simulink model "kalman_scattering_based_fv"  (R2020b)
settings: Solver=ode45  StartTime=0.0  StopTime=30  RelTol=1e-3
values from neighbouring files (symbols this model uses):
  A = [1 Ts ... (first row only)    [kalman_hw6_main_fv.m]
  Amp = 0.3    [kalman_hw6_main_fv.m]
  b = 1    [kalman_hw6_main_fv.m]
  Be = 20    [kalman_hw6_main_fv.m]
  Bh = 1.5    [kalman_hw6_main_fv.m]
  Bs = 50    [kalman_hw6_main_fv.m]
  C = [1 0]    [kalman_hw6_main_fv.m]
  delay = 10    [kalman_hw6_main_fv.m]
  Dh = 8    [kalman_hw6_main_fv.m]
  Dm = 0    [kalman_hw6_main_fv.m]
  Ds = 0    [kalman_hw6_main_fv.m]
  Fc_lp = 5    [kalman_hw6_main_fv.m]
  Fc_sin = 0.1    [kalman_hw6_main_fv.m]
  Fc_wave = 8    [kalman_hw6_main_fv.m]
  Je = 0    [kalman_hw6_main_fv.m]
  Jh = 0    [kalman_hw6_main_fv.m]
  Ke = 210    [kalman_hw6_main_fv.m]
  Kh = 0.1    [kalman_hw6_main_fv.m]
  Ks = 60    [kalman_hw6_main_fv.m]
  Mm = 0.5    [kalman_hw6_main_fv.m]
  Ms = 2    [kalman_hw6_main_fv.m]
  Ph = 1    [kalman_hw6_main_fv.m]
  posNoiseVar = 0.0001    [kalman_hw6_main_fv.m]
  R_m = 1    [kalman_hw6_main_fv.m]
  R_s = 1    [kalman_hw6_main_fv.m]
  torqueNoiseVar = 0.01    [kalman_hw6_main_fv.m]
  Ts = 0.001    [kalman_hw6_main_fv.m]
  xe = 0.5    [kalman_hw6_main_fv.m]
undefined symbols (not defined in the file or in its folder): DiscIntNeverNeededParam, Discrete, Time
libraries: simulink x4, ctrlSharedLib x2
settings Model: Creator=nicol  LastModifiedBy=nicol

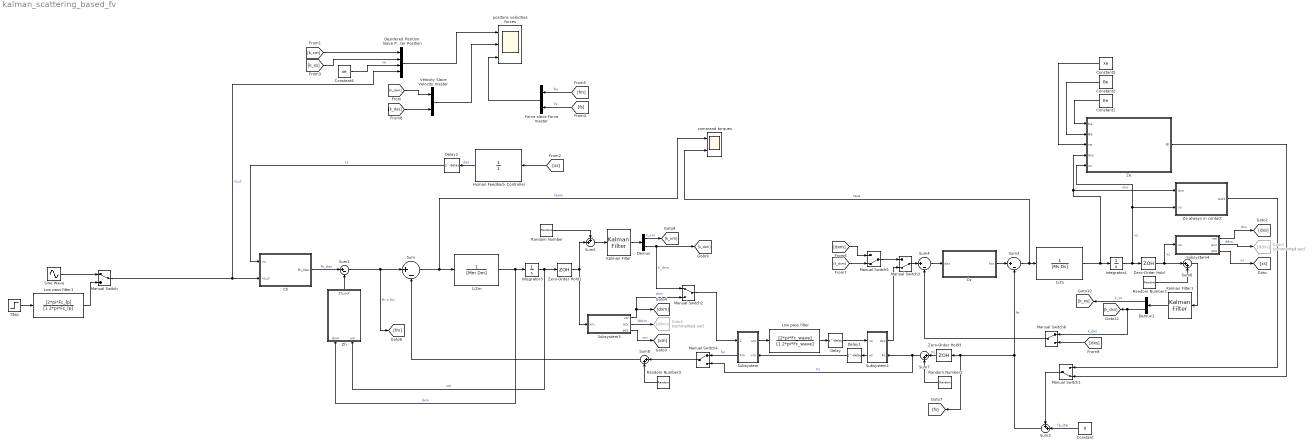
== system kalman_scattering_based_fv ==
  1/Zm : TransferFcn  Denominator=[Mm Dm]
  1/Zs : TransferFcn  Denominator=[Ms Ds]
  Ch : Subsystem
  Constant : Constant  Value=0
  Constant1 : Constant  Value=Ke
  Constant2 : Constant  Value=Be
  Constant3 : Constant  Value=xe
  Constant4 : Constant  Value=xe
  Cs : Subsystem
  Delay : Delay  DelayLength=delay  SampleTime=Ts
  Delay1 : Delay  DelayLength=delay  SampleTime=Ts
  Delay2 : Delay  DelayLength=delay  SampleTime=Ts
  Demux : Demux  Outputs=2
  Demux1 : Demux  Outputs=2
  Desidered Position Slave Position Master Position : Mux
  Force slave Force master : Mux  Inputs=2
  Goto2 : Goto  Commented=on  GotoTag=ddxs
  Goto5 : Goto  Commented=on  GotoTag=ddxm
  Human Feedback Controller : TransferFcn  Denominator=[1]
  Integrator3 : Integrator
  Integrator4 : Integrator
  Kalman Filter : ctrlSharedLib/Kalman Filter  TimeDomain=Discrete-Time  UseCurrentEstimator=on  ModelSource=Individual A, B, C, D matrices  ModelSourceVariable=ss(0.95,1,0,0,Ts)  A=A  B=1  C=C  D=0  NumberOfStates=1  NumberOfInputs=1  NumberOfOutputs=1  InitialEstimateSource=Dialog  X0=0  P0=10  UseK=off  UseGH=off  NumberOfProcessNoiseInputs=1  G=1  TimeInvariantG=on  H=0  TimeInvariantH=on  Q=Q_m  TimeInvariantQ=on  R=R_m  TimeInvariantR=on  N=0  TimeInvariantN=on  AddInputPort=off  AddEnablePort=off  OutputEstimatedY=off  OutputP=off  Ts=Ts
  Kalman Filter1 : ctrlSharedLib/Kalman Filter  TimeDomain=Discrete-Time  UseCurrentEstimator=on  ModelSource=Individual A, B, C, D matrices  ModelSourceVariable=ss(0.95,1,0,0,Ts)  A=A  B=1  C=C  D=0  NumberOfStates=1  NumberOfInputs=1  NumberOfOutputs=1  InitialEstimateSource=Dialog  X0=0  P0=10  UseK=off  UseGH=off  NumberOfProcessNoiseInputs=1  G=1  TimeInvariantG=on  H=0  TimeInvariantH=on  Q=Q_s  TimeInvariantQ=on  R=R_s  TimeInvariantR=on  N=0  TimeInvariantN=on  AddInputPort=off  AddEnablePort=off  OutputEstimatedY=off  OutputP=off  Ts=Ts
  Low pass filter : TransferFcn  Numerator=[2*pi*Fc_wave]  Denominator=[1 2*pi*Fc_wave]
  Low pass filter1 : TransferFcn  Numerator=[2*pi*Fc_lp]  Denominator=[1 2*pi*Fc_lp]
  Manual Switch{,2,4,6} (4 alike) : ManualSwitch
  Manual Switch1 : ManualSwitch  CurrentSetting=0
  Manual Switch3 : ManualSwitch  CurrentSetting=0
  Manual Switch5 : ManualSwitch  CurrentSetting=0
  Random Number : RandomNumber  Variance=posNoiseVar  SampleTime=Ts
  Random Number1 : RandomNumber  Variance=posNoiseVar  SampleTime=Ts
  Random Number2 : RandomNumber  Variance=torqueNoiseVar  SampleTime=Ts
  Random Number3 : RandomNumber  Variance=torqueNoiseVar  SampleTime=Ts
  Sine Wave : Sin  Amplitude=Amp  Frequency=2*pi*Fc_sin  SampleTime=0
  Step : Step  Time=Amp  After=Amp  SampleTime=0
  Subsystem : Subsystem
      settings: PortSchema="{\"entries\":[{\"content\":{\"sides\":[{\"content\":{\"connectorIds\":[\"In1\",\"Out2\"]},\"type\":\"ConnectorPlacement.EquallySpacedRectSide\",\"uuid\":\"82be490b-f4e1-4469-8bd6-488a0e070f91\"},{\"content\":{\"connectorIds\":[\"Out1\",\"In2\"],\"side\":\"RIGHT\"},\"type\":\"ConnectorPlacement.EquallySpacedRectSide\",\"uuid\":\"c4a13bf6-21c5-475e-be70-cb3636e820b8\"},{\"content\":{\"connectorIds\":[],\"side\":\"TOP\"},\"type\":\"ConnectorPlacement.EquallySpacedRectSide\",\"uuid\":\"239945ea-98d9-43ca-9337-d0acd489fa2c\"},{\"content\":{\"connectorIds\":[],\"side\":\"HIDDEN\"},\"type\":\"ConnectorPlacement.EquallySpacedRectSide\",\"uuid\":\"ab55d6c9-2d6b-496a-b62d-f74546630c92\"}]},\"type\":\"ConnectorPlacement.EquallySpacedConnector\",\"uuid\":\"f2ee4140-76ed-4153-9f7f-3580e67d072a\"}],\"packageUris\":[\"http://schema.mathworks.com/mf0/Connector/R2020b\"],\"version\":\"1.0\"}"
  Subsystem1 : Subsystem
      settings: PortSchema="{\"entries\":[{\"content\":{\"sides\":[{\"content\":{\"connectorIds\":[\"In1\",\"Out2\"]},\"type\":\"ConnectorPlacement.EquallySpacedRectSide\",\"uuid\":\"82be490b-f4e1-4469-8bd6-488a0e070f91\"},{\"content\":{\"connectorIds\":[\"Out1\",\"In2\"],\"side\":\"RIGHT\"},\"type\":\"ConnectorPlacement.EquallySpacedRectSide\",\"uuid\":\"c4a13bf6-21c5-475e-be70-cb3636e820b8\"},{\"content\":{\"connectorIds\":[],\"side\":\"TOP\"},\"type\":\"ConnectorPlacement.EquallySpacedRectSide\",\"uuid\":\"239945ea-98d9-43ca-9337-d0acd489fa2c\"},{\"content\":{\"connectorIds\":[],\"side\":\"HIDDEN\"},\"type\":\"ConnectorPlacement.EquallySpacedRectSide\",\"uuid\":\"ab55d6c9-2d6b-496a-b62d-f74546630c92\"}]},\"type\":\"ConnectorPlacement.EquallySpacedConnector\",\"uuid\":\"f2ee4140-76ed-4153-9f7f-3580e67d072a\"}],\"packageUris\":[\"http://schema.mathworks.com/mf0/Connector/R2020b\"],\"version\":\"1.0\"}"
  Subsystem3 : Subsystem
  Subsystem4 : Subsystem
  Sum{,1..2,4} (4 alike) : Sum  Inputs=|+-
  Sum3 : Sum  Inputs=++|
  Sum5 : Sum  Inputs=++|
  Sum6 : Sum  Inputs=|++
  Sum7 : Sum  Inputs=|++
  Sum8 : Sum  Inputs=|++
  Velocity Slave Velocity master : Mux  Inputs=2
  Ze : MATLAB Function  TreatAsAtomicUnit=on
  Ze always in contact : Subsystem
  Zero-Order Hold : ZeroOrderHold  SampleTime=Ts
  Zero-Order Hold1 : ZeroOrderHold  SampleTime=Ts
  Zero-Order Hold3 : ZeroOrderHold  SampleTime=Ts
  Zh : Subsystem
  command torques : Scope  NumInputPorts=2
  "positons velocities forces " : Scope  NumInputPorts=3
  wires:
  Ch/1(fh_star) -> Sum1/1  "fh_star"
  Zh/1(Zh_out) -> Sum1/2
  1/Zm/1 -> Zh/1(dxm), Integrator3/1  "dxm"
  Sum1/1 -> Sum/1, [fm]  "fh = fm"
  Cs/1(fcs) -> Sum2/1
  1/Zs/1 -> Integrator4/1, Ze always in contact/1(dxs), Ze/4(dxs)  "dxs"
  Sum2/1 -> 1/Zs/1, command torques/2  "taus"
  Ze/1(fE) -> Manual Switch1/2
  Sum3/1 -> [fs], Zero-Order Hold3/1, Sum2/2  "fe"
  Constant/1 -> Sum3/2  "fe_star"
  Constant1/1 -> Ze/1(Ke)
  Constant2/1 -> Ze/2(Be)
  Constant3/1 -> Ze/3(xe)
  Integrator4/1 -> Ze/5(xs), Ze always in contact/2(xs), Zero-Order Hold/1  "xs"
  Manual Switch1/1 -> Sum3/1
  Ze always in contact/1(out1) -> Manual Switch1/1
  Sum/1 -> command torques/1, 1/Zm/1  "taum"
  Velocity Slave Velocity master/1 -> "positons velocities forces "/2
  Desidered Position Slave Position Master Position/1 -> "positons velocities forces "/1
  Sum4/1 -> Cs/1(dxs)
  Manual Switch/1 -> Desidered Position Slave Position Master Position/4, Ch/2(xs_d)  "xs_d"
  Subsystem3/1(vel) -> [dxm], Manual Switch2/2  "dxm"
  Subsystem3/3(pos) -> [xm]  "xm"
  Integrator3/1 -> Zero-Order Hold1/1, Zh/2(xm)  "xm"
  Subsystem3/2(acc) -> Goto5/1  "ddxm"
  Subsystem4/2(acc) -> Goto2/1  "ddxs"
  Subsystem4/1(vel) -> [dxs]  "dxs"
  Subsystem4/3(pos) -> [xs]  "xs"
  Zero-Order Hold/1 -> Sum6/1, Subsystem4/1(xs)  "xs"
  [xs] -> Human Feedback Controller/1
  Delay2/1 -> Ch/1(xs)  "xs"
  Delay1/1 -> Subsystem/2(vm)
  Delay/1 -> Subsystem1/1(vs)
  Subsystem/1(um) -> Low pass filter/1
  Subsystem1/2(us) -> Delay1/1
  Human Feedback Controller/1 -> Delay2/1  "dxs"
  Zero-Order Hold1/1 -> Subsystem3/1(xm), Sum5/2
  Sine Wave/1 -> Manual Switch/1
  [k_dxm] -> Velocity Slave Velocity master/1
  [k_xm] -> Desidered Position Slave Position Master Position/1
  [k_xs] -> Desidered Position Slave Position Master Position/2
  Constant4/1 -> Desidered Position Slave Position Master Position/3  "xe"
  Subsystem1/1(dxs) -> Manual Switch3/2
  Low pass filter/1 -> Delay/1
  Step/1 -> Low pass filter1/1
  [k_dxs] -> Velocity Slave Velocity master/2
  Low pass filter1/1 -> Manual Switch/2
  Force slave Force master/1 -> "positons velocities forces "/3
  [fs] -> Force slave Force master/2  "fs"
  [fm] -> Force slave Force master/1  "fm"
  Manual Switch3/1 -> Sum4/1
  Subsystem/2(Fm) -> Manual Switch4/1  "fm"
  Random Number/1 -> Sum5/1
  Sum5/1 -> Kalman Filter/1
  Kalman Filter/1 -> Demux/1
  Demux/1 -> [k_xm]  "k_xm"
  Demux/2 -> Manual Switch2/1, [k_dxm]  "k_dxm"
  Manual Switch2/1 -> Subsystem/1(dxm)
  [dxm] -> Manual Switch5/1
  [k_dxm] -> Manual Switch5/2
  Manual Switch5/1 -> Manual Switch3/1
  Random Number1/1 -> Sum6/2
  Demux1/2 -> Manual Switch6/1, [k_dxs]  "k_dxs"
  Kalman Filter1/1 -> Demux1/1
  Demux1/1 -> [k_xs]  "k_xs"
  Sum6/1 -> Kalman Filter1/1
  [dxs] -> Manual Switch6/2
  Manual Switch6/1 -> Sum4/2
  Random Number2/1 -> Sum7/2
  Zero-Order Hold3/1 -> Sum7/1  "Fs"
  Sum7/1 -> Manual Switch4/2, Subsystem1/2(Fs)  "Fs"
  Random Number3/1 -> Sum8/2
  Manual Switch4/1 -> Sum8/1
  Sum8/1 -> Sum/2

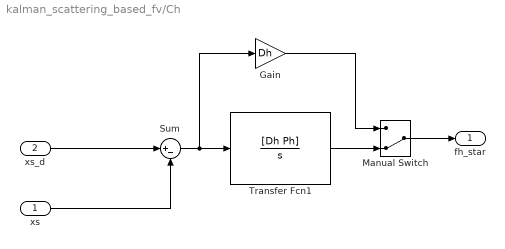
== system kalman_scattering_based_fv/Ch ==
  xs : Inport
  xs_d : Inport  Port=2
  Gain : Gain  Gain=Dh
  Manual Switch : ManualSwitch  CurrentSetting=0
  Sum : Sum  Inputs=|+-
  Transfer Fcn1 : TransferFcn  Numerator=[Dh Ph]  Denominator=[1 0]
  fh_star : Outport
  wires:
  xs/1 -> Sum/2
  Sum/1 -> Gain/1, Transfer Fcn1/1
  xs_d/1 -> Sum/1
  Gain/1 -> Manual Switch/1
  Transfer Fcn1/1 -> Manual Switch/2
  Manual Switch/1 -> fh_star/1

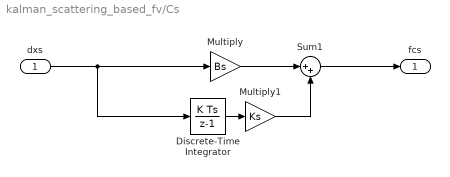
== system kalman_scattering_based_fv/Cs ==
  dxs : Inport
  Discrete-Time Integrator : DiscreteIntegrator  SampleTime=-1  ICPrevOutput=DiscIntNeverNeededParam  ICPrevScaledInput=DiscIntNeverNeededParam
  Multiply : Gain  Gain=Bs
  Multiply1 : Gain  Gain=Ks
  Sum1 : Sum  Inputs=|++
  fcs : Outport
  wires:
  dxs/1 -> Discrete-Time Integrator/1, Multiply/1
  Multiply1/1 -> Sum1/2
  Multiply/1 -> Sum1/1
  Sum1/1 -> fcs/1
  Discrete-Time Integrator/1 -> Multiply1/1

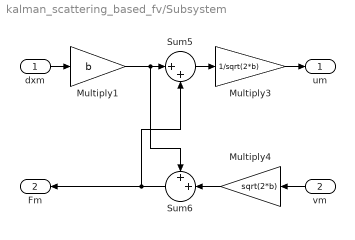
== system kalman_scattering_based_fv/Subsystem ==
  dxm : Inport
  vm : Inport  Port=2
  Multiply1 : Gain  Gain=b
  Multiply3 : Gain  Gain=1/sqrt(2*b)
  Multiply4 : Gain  Gain=sqrt(2*b)
  Sum5 : Sum  Inputs=|++
  Sum6 : Sum  Inputs=++|
  um : Outport
  Fm : Outport  Port=2
  wires:
  Sum6/1 -> Fm/1, Sum5/2
  Multiply1/1 -> Sum6/1, Sum5/1
  Sum5/1 -> Multiply3/1
  Multiply4/1 -> Sum6/2
  vm/1 -> Multiply4/1
  Multiply3/1 -> um/1
  dxm/1 -> Multiply1/1

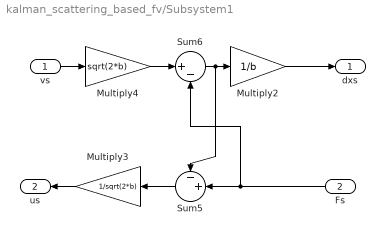
== system kalman_scattering_based_fv/Subsystem1 ==
  vs : Inport
  Fs : Inport  Port=2
  Multiply2 : Gain  Gain=1/b
  Multiply3 : Gain  Gain=1/sqrt(2*b)
  Multiply4 : Gain  Gain=sqrt(2*b)
  Sum5 : Sum  Inputs=-+|
  Sum6 : Sum  Inputs=|+-
  dxs : Outport
  us : Outport  Port=2
  wires:
  Sum6/1 -> Sum5/1, Multiply2/1
  Sum5/1 -> Multiply3/1
  Fs/1 -> Sum5/2, Sum6/2
  vs/1 -> Multiply4/1
  Multiply2/1 -> dxs/1
  Multiply3/1 -> us/1
  Multiply4/1 -> Sum6/1

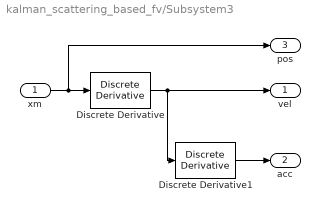
== system kalman_scattering_based_fv/Subsystem3 ==
  xm : Inport
  Discrete Derivative : simulink/Discrete/Discrete Derivative  gainval=1.0  ICPrevScaledInput=0.0  OutMin=[]  OutMax=[]  OutDataType=fixdt(1, 16)  OutScaling=2^-10  DoSatur=off
  Discrete Derivative1 : simulink/Discrete/Discrete Derivative  gainval=1.0  ICPrevScaledInput=0.0  OutMin=[]  OutMax=[]  OutDataType=fixdt(1, 16)  OutScaling=2^-10  DoSatur=off
  vel : Outport
  acc : Outport  Port=2
  pos : Outport  Port=3
  wires:
  xm/1 -> pos/1, Discrete Derivative/1
  Discrete Derivative/1 -> Discrete Derivative1/1, vel/1
  Discrete Derivative1/1 -> acc/1

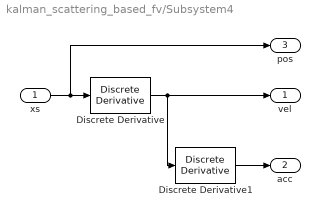
== system kalman_scattering_based_fv/Subsystem4 ==
  xs : Inport
  Discrete Derivative : simulink/Discrete/Discrete Derivative  gainval=1.0  ICPrevScaledInput=0.0  OutMin=[]  OutMax=[]  OutDataType=fixdt(1, 16)  OutScaling=2^-10  DoSatur=off
  Discrete Derivative1 : simulink/Discrete/Discrete Derivative  gainval=1.0  ICPrevScaledInput=0.0  OutMin=[]  OutMax=[]  OutDataType=fixdt(1, 16)  OutScaling=2^-10  DoSatur=off
  vel : Outport
  acc : Outport  Port=2
  pos : Outport  Port=3
  wires:
  xs/1 -> pos/1, Discrete Derivative/1
  Discrete Derivative/1 -> Discrete Derivative1/1, vel/1
  Discrete Derivative1/1 -> acc/1

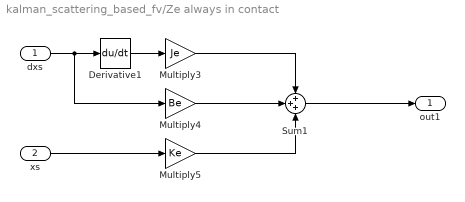
== system kalman_scattering_based_fv/Ze always in contact ==
  dxs : Inport
  xs : Inport  Port=2
  Derivative1 : Derivative
  Multiply3 : Gain  Gain=Je
  Multiply4 : Gain  Gain=Be
  Multiply5 : Gain  Gain=Ke
  Sum1 : Sum  Inputs=+++
  out1 : Outport
  wires:
  Sum1/1 -> out1/1
  Multiply4/1 -> Sum1/2
  Multiply5/1 -> Sum1/3
  dxs/1 -> Multiply4/1, Derivative1/1
  Derivative1/1 -> Multiply3/1
  xs/1 -> Multiply5/1
  Multiply3/1 -> Sum1/1

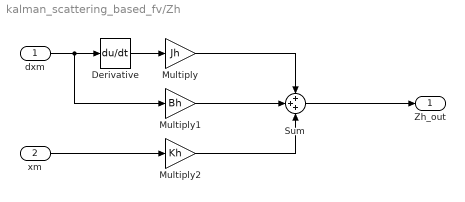
== system kalman_scattering_based_fv/Zh ==
  dxm : Inport
  xm : Inport  Port=2
  Derivative : Derivative
  Multiply : Gain  Gain=Jh
  Multiply1 : Gain  Gain=Bh
  Multiply2 : Gain  Gain=Kh
  Sum : Sum  Inputs=+++
  Zh_out : Outport
  wires:
  dxm/1 -> Multiply1/1, Derivative/1
  Derivative/1 -> Multiply/1
  Sum/1 -> Zh_out/1
  xm/1 -> Multiply2/1
  Multiply1/1 -> Sum/2
  Multiply/1 -> Sum/1
  Multiply2/1 -> Sum/3

== matlab function kalman_scattering_based_fv/Ze ==
  data: Ke input; fE output; Be input; xe input; dxs input; xs input
function fE = environment(Ke, Be, xe, dxs, xs)
if(xs > xe)
    fE = Ke*(xs - xe) + Be*dxs;
else
    fE=0;
end
